simulink model "MultiADCTest"  (R2023b)
settings: Solver=VariableStepAuto  StartTime=0.0  StopTime=5e-3  RelTol=1e-3
settings Model: Creator=rlschie  LastModifiedBy=rlschie

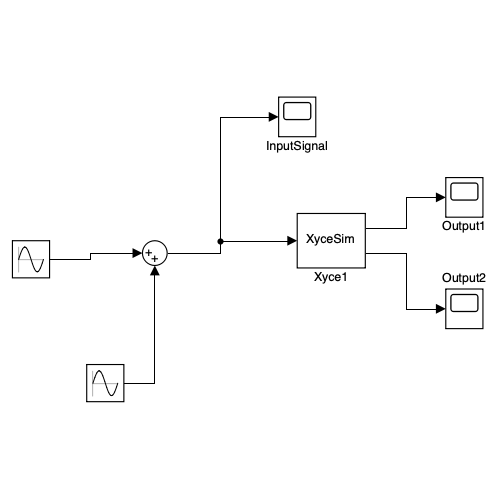
[thumbnail: Simulink's stored preview of the top-level diagram]
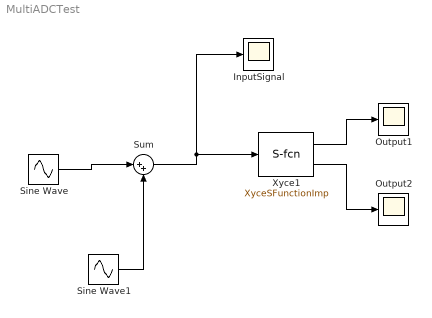
== system MultiADCTest ==
  InputSignal : Scope
  Output1 : Scope
  Output2 : Scope
  Sine Wave : Sin  Amplitude=5  Frequency=5e3  SampleTime=0
  Sine Wave1 : Sin  Amplitude=3  Frequency=2e4  SampleTime=0
  Sum : Sum  Inputs=|++
  Xyce1 : M-S-Function  FunctionName=XyceSFunctionImp  Parameters=XyceInputFileName,WorkingDirectory,NumberOfInputs,NumberOfOutputs,InputNames,OutputNames  mask{XyceNumberOfOutputPorts=0, XyceNumberOfInputPorts=0, XyceOutputPortNames=, XyceInputPortNames=, WorkingDirectory=/Users/rlschie/src/XyceDevelopment/INSTALL/share/SimulinkExamples/, XyceInputFileName=MultiADCTest.cir, NumberOfInputs=1, NumberOfOutputs=2, InputNames={ '1', 'YDAC!DACDRIVER1' }, OutputNames={ '1', 'YADC!ADCLOW'; '2', 'YADC!ADCHIGH' }}
      mask prompts: XyceNumberOfOutputPorts "Xyce Number Of Outputs"; XyceNumberOfInputPorts "Xyce Number Of Inputs"; XyceOutputPortNames "Xyce Output Port Names"; XyceInputPortNames "Xyce Input Port Names"; WorkingDirectory "Working Directory"; XyceInputFileName "Xyce Input Filename"; NumberOfInputs "Number of Inputs"; NumberOfOutputs "Number of Outputs"; InputNames "Input Names"; OutputNames "Output Names"
      mask DialogControl SelectXyceInputFileButton Prompt: Select Xyce Input File
      mask DialogControl ScanXyceInputFileButton Prompt: Scan Xyce Input File
      mask DialogControl ResetForm Prompt: Reset
      mask DialogControl AddInputLineButton Prompt: Add Line
      mask DialogControl RemoveInputLineButton Prompt: Remove Line
      mask DialogControl AddOutputLineButton Prompt: Add Line
      mask DialogControl RemoveOutputLineButton Prompt: Remove Line
      mask Display: disp('XyceSim');
  wires:
  Sine Wave/1 -> Sum/1
  Sine Wave1/1 -> Sum/2
  Sum/1 -> InputSignal/1, Xyce1/1
  Xyce1/1 -> Output1/1
  Xyce1/2 -> Output2/1
